simulink model "b_absorption_chiller_Yazaki_WFC_SC5_R2012a"  (Simulink 7.6)
settings: Solver=ode45  StartTime=0.0  StopTime=5000  FixedStep=1  RelTol=1e-3
PreLoadFcn:
  | load Yazaki_KF.mat;
values from neighbouring files (symbols this model uses):
  WFC_q_cold = [7.01442779481 14.9293699635 19.0103 4.77399164271 12.8469320096 16.2646 2.68674680792 10.4033145599 13.7100752403 6.86044435277 15.261380912 20.4077 ... (27 elements, 3x3x3)]    [Yazaki_KF.mat]
  WFC_q_hot = [11.58810793 12.70101443 13.76292339 14.78464775 15.7778999 16.75684251 17.73693962 18.73523022 19.7725001 20.87266321 21.46134147 22.12214918 ... (171 elements, 19x3x3)]    [Yazaki_KF.mat]
  WFC_q_recooling = [17.7490465324 34.7262277405 45.9087 12.9282238624 30.2579685905 40.8416 8.70035517453 25.0503537415 35.7528254726 17.2271014606 35.4257858178 48.632 ... (27 elements, 3x3x3)]    [Yazaki_KF.mat]
undefined symbols (not defined in the file or in its folder): A, B, C, Dd
settings Model: Creator=Simulation  LastModifiedBy=fabian.ille
settings DebuggingCC: FcnCallInpInsideContextMsg=Enable All
settings GRTTargetCC: CombineOutputUpdateFcns=on

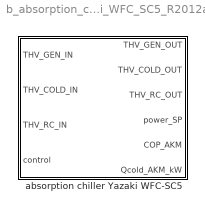
== system b_absorption_chiller_Yazaki_WFC_SC5_R2012a ==
  absorption chiller Yazaki WFC-SC5 : Subsystem
      mask Type: absorption chiller Yazaki WFC-SC5
      mask Description:
      | This block calculates the capacities and cop of the absorption chiller Yazaki WFC-SC5 (nominal cooling capacity: 17.6 kW, nominal COP: 0.7) based on measured curves.
      | Measurement range:
      | T_HT_IN 70 .. 88 °C, T_MT_IN 29 .. 33 °C, T_NT_IN 11 .. 14 °C
      | Outside of this range the lookup-tables extrapolate.
      | 
      | It is only valid for the following volumeflows:
      | HT: 4320 l/h, MT: 9180 l/h, NT: 2770 l/h
      | 
      | It includes a dynamic start-up behaviour with a dead time of the cooling capacity and capacities in all cycles.
      | Additionally the power of the solution pump is given out.
      mask Help: eval('helpcarnot')

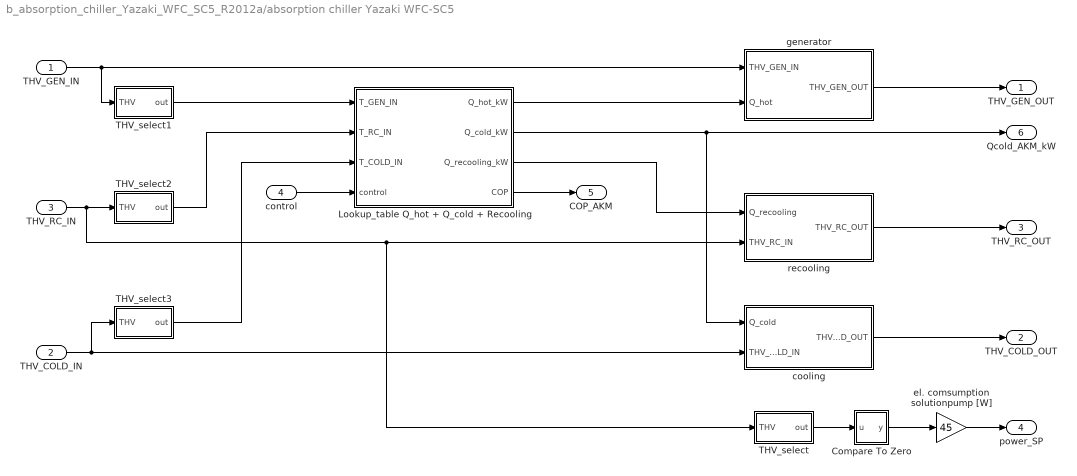
== system b_absorption_chiller_Yazaki_WFC_SC5_R2012a/absorption chiller Yazaki WFC-SC5 ==
  THV_GEN_IN : Inport
  THV_COLD_IN : Inport  Port=2
  THV_RC_IN : Inport  Port=3
  control : Inport  Port=4
  Compare To Zero : Subsystem  mask(Compare To Zero){relop=>, LogicOutDataTypeMode=uint8, ZeroCross=on}
      mask prompts: relop "Operator:"; LogicOutDataTypeMode "Output data type mode:"; ZeroCross "Enable zero-crossing detection"
      mask help: Determine how a signal compares to zero.
      mask init:
      | blkName = gcb;
      | 
      | if strcmp(get_param(gcbh,'LogicOutDataTypeMode'),'boolean')
      | 	setValue = 'Boolean';
      | else
      |     setValue = 'Specify via dialog';
      | end
      | 
      | set_param([blkName,'/Compare'],'relop',relop, ...
      | 	'LogicOutDataTypeMode', setValue, 'ZeroCross', ZeroCross);
      mask StyleString: popup(==|~=|<|<=|>=|>),popup(uint8|boolean),checkbox
      mask CallbackString: ||sl('zeroCrossEnable', gcbh);
      mask Display: disp([relop,' 0'])
  Lookup_table Q_hot + Q_cold + Recooling : Subsystem  TreatAsAtomicUnit=on
  THV_select : Subsystem  mask(select from THV){f=off, t=off, m=on, p=off, id=off, mix=off, d=off, dpcon=off, dplin=off, dpqua=off}
      mask prompts: f "flow identifier"; t "temperature [degree centigrade]"; m "massflow [kg/s]"; p "pressure [Pa]"; id "fluid ID (1 = water, 2 = air, 3 = cotton oil, 4 = water-glycol)"; mix "fluid mix"; d "diameter [m]"; dpcon "constant press. drop"; dplin "linear pressure drop"; dpqua "quadratic pressure drop"
      mask help: Selects the ticked values from the thermo hydraulic vector.
      mask init:
      | v=[];
      | if (f)
      |     v  = [1];
      | end
      | if (t)
      |     v  = [v 2];
      | end
      | if (m)
      |     v= [v 3];
      | end
      | if (p)
      |     v = [v 4];
      | end
      | if (id)
      |     v = [v 5];
      | end
      | if (mix)
      |     v = [v 6];
      | end
      | if (d)
      |     v = [v 7];
      | end
      | if (dpcon)
      |     v = [v 8];
      | end
      | if (dplin)
      |     v = [v 9];
      | end
      | if (dpqua)
      |     v = [v 10];
      | end
      mask Help: eval('man(''THV_select'')')
  THV_select1 : Subsystem  mask(select from THV){f=off, t=on, m=off, p=off, id=off, mix=off, d=off, dpcon=off, dplin=off, dpqua=off}
      mask prompts: f "flow identifier"; t "temperature [degree centigrade]"; m "massflow [kg/s]"; p "pressure [Pa]"; id "fluid ID (1 = water, 2 = air, 3 = cotton oil, 4 = water-glycol)"; mix "fluid mix"; d "diameter [m]"; dpcon "constant press. drop"; dplin "linear pressure drop"; dpqua "quadratic pressure drop"
      mask help: Selects the ticked values from the thermo hydraulic vector.
      mask init: same as b_absorption_chiller_Yazaki_WFC_SC5_R2012a/absorption chiller Yazaki WFC-SC5/THV_select
      mask Help: eval('man(''THV_select'')')
  THV_select2 : Subsystem  mask(select from THV){f=off, t=on, m=off, p=off, id=off, mix=off, d=off, dpcon=off, dplin=off, dpqua=off}
      mask prompts: f "flow identifier"; t "temperature [degree centigrade]"; m "massflow [kg/s]"; p "pressure [Pa]"; id "fluid ID (1 = water, 2 = air, 3 = cotton oil, 4 = water-glycol)"; mix "fluid mix"; d "diameter [m]"; dpcon "constant press. drop"; dplin "linear pressure drop"; dpqua "quadratic pressure drop"
      mask help: Selects the ticked values from the thermo hydraulic vector.
      mask init: same as b_absorption_chiller_Yazaki_WFC_SC5_R2012a/absorption chiller Yazaki WFC-SC5/THV_select
      mask Help: eval('man(''THV_select'')')
  THV_select3 : Subsystem  mask(select from THV){f=off, t=on, m=off, p=off, id=off, mix=off, d=off, dpcon=off, dplin=off, dpqua=off}
      mask prompts: f "flow identifier"; t "temperature [degree centigrade]"; m "massflow [kg/s]"; p "pressure [Pa]"; id "fluid ID (1 = water, 2 = air, 3 = cotton oil, 4 = water-glycol)"; mix "fluid mix"; d "diameter [m]"; dpcon "constant press. drop"; dplin "linear pressure drop"; dpqua "quadratic pressure drop"
      mask help: Selects the ticked values from the thermo hydraulic vector.
      mask init: same as b_absorption_chiller_Yazaki_WFC_SC5_R2012a/absorption chiller Yazaki WFC-SC5/THV_select
      mask Help: eval('man(''THV_select'')')
  cooling : Subsystem
  el. comsumption solutionpump [W] : Gain  Gain=45
  generator : Subsystem
  recooling : Subsystem
  THV_GEN_OUT : Outport
  THV_COLD_OUT : Outport  Port=2
  THV_RC_OUT : Outport  Port=3
  power_SP : Outport  Port=4
  COP_AKM : Outport  Port=5
  Qcold_AKM_kW : Outport  Port=6
  wires:
  THV_COLD_IN/1 -> THV_select3/1(THV), cooling/2(THV_COLD_IN)
  THV_GEN_IN/1 -> THV_select1/1(THV), generator/1(THV_GEN_IN)
  generator/1(THV_GEN_OUT) -> THV_GEN_OUT/1
  THV_RC_IN/1 -> THV_select2/1(THV), THV_select/1(THV), recooling/2(THV_RC_IN)
  THV_select2/1(out) -> Lookup_table Q_hot + Q_cold + Recooling/2(T_RC_IN)
  recooling/1(THV_RC_OUT) -> THV_RC_OUT/1
  cooling/1(THV_COLD_OUT) -> THV_COLD_OUT/1
  control/1 -> Lookup_table Q_hot + Q_cold + Recooling/4(control)
  THV_select3/1(out) -> Lookup_table Q_hot + Q_cold + Recooling/3(T_COLD_IN)
  Lookup_table Q_hot + Q_cold + Recooling/2(Q_cold_kW) -> cooling/1(Q_cold), Qcold_AKM_kW/1
  Lookup_table Q_hot + Q_cold + Recooling/1(Q_hot_kW) -> generator/2(Q_hot)
  Lookup_table Q_hot + Q_cold + Recooling/3(Q_recooling_kW) -> recooling/1(Q_recooling)
  el. comsumption solutionpump [W]/1 -> power_SP/1
  THV_select/1(out) -> Compare To Zero/1(u)
  Compare To Zero/1(y) -> el. comsumption solutionpump [W]/1
  THV_select1/1(out) -> Lookup_table Q_hot + Q_cold + Recooling/1(T_GEN_IN)
  Lookup_table Q_hot + Q_cold + Recooling/4(COP) -> COP_AKM/1

== system b_absorption_chiller_Yazaki_WFC_SC5_R2012a/absorption chiller Yazaki WFC-SC5/Compare To Zero ==
  u : Inport
  Compare : RelationalOperator  Operator=>  OutDataTypeStr=fixdt(0, 8)
  Constant : Constant  DisableCoverage=on  Value=0  OutDataTypeStr=Inherit: Inherit via back propagation  PreserveConstantTs=on
  y : Outport
  wires:
  Constant/1 -> Compare/2
  u/1 -> Compare/1
  Compare/1 -> y/1

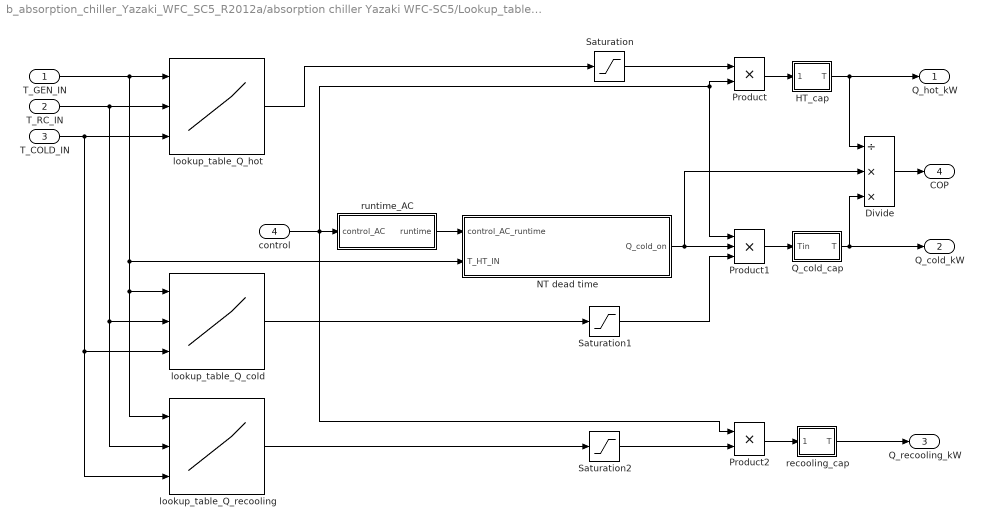
== system b_absorption_chiller_Yazaki_WFC_SC5_R2012a/absorption chiller Yazaki WFC-SC5/Lookup_table Q_hot + Q_cold + Recooling ==
  T_GEN_IN : Inport
  T_RC_IN : Inport  Port=2
  T_COLD_IN : Inport  Port=3
  control : Inport  Port=4
  Divide : Product  Inputs=/**
  HT_cap : Subsystem  mask(capacity){NTU=0.0464, Tini=0}
      mask prompts: NTU "heat transfer / heat capacity NTU (k*A/(m*cp))"; Tini "initial temperature [degree centigrade]"
      mask help: The block introduces a capacity of the component. It can be used to break an algebraic loop.
      mask Help: eval('man(''capacity'')')
  NT dead time : Stateflow chart  TreatAsAtomicUnit=on
  Product : Product  RndMeth=Zero
  Product1 : Product  Inputs=3  RndMeth=Zero
  Product2 : Product  RndMeth=Zero
  Q_cold_cap : Subsystem  mask(capacity){NTU=0.0191, Tini=0}
      mask prompts: NTU "heat transfer / heat capacity NTU (k*A/(m*cp))"; Tini "initial temperature [degree centigrade]"
      mask help: The block introduces a capacity of the component. It can be used to break an algebraic loop.
      mask Help: eval('man(''capacity'')')
  Saturation : Saturate  UpperLimit=inf  LowerLimit=0
  Saturation1 : Saturate  UpperLimit=inf  LowerLimit=0
  Saturation2 : Saturate  UpperLimit=inf  LowerLimit=0
  lookup_table_Q_cold : Lookup_n-D  NumberOfTableDimensions=3  BreakpointsForDimension1=[70,79,88]  BreakpointsForDimension2=[29,31,33]  BreakpointsForDimension3=[11,12.5,14]  BreakpointsForDimension4=[1:2]  Table=WFC_q_cold  InputSameDT=on
  lookup_table_Q_hot : Lookup_n-D  NumberOfTableDimensions=3  BreakpointsForDimension1=[70:1:88]  BreakpointsForDimension2=[29,31,33]  BreakpointsForDimension3=[11,12.5,14]  BreakpointsForDimension4=[1:2]  Table=WFC_q_hot  InputSameDT=on
  lookup_table_Q_recooling : Lookup_n-D  NumberOfTableDimensions=3  BreakpointsForDimension1=[70,79,88]  BreakpointsForDimension2=[29,31,33]  BreakpointsForDimension3=[11,12.5,14]  BreakpointsForDimension4=[1:2]  Table=WFC_q_recooling  InputSameDT=on
  recooling_cap : Subsystem  mask(capacity){NTU=0.0096, Tini=0}
      mask prompts: NTU "heat transfer / heat capacity NTU (k*A/(m*cp))"; Tini "initial temperature [degree centigrade]"
      mask help: The block introduces a capacity of the component. It can be used to break an algebraic loop.
      mask Help: eval('man(''capacity'')')
  runtime_AC : Subsystem  TreatAsAtomicUnit=on
      mask Description: This block counts the time if input is set to one, it stops counting if input is zero and continues when input rises to one again.
      mask Help: eval('filetest (''manual.htm#count_working_time'')')
  Q_hot_kW : Outport
  Q_cold_kW : Outport  Port=2
  Q_recooling_kW : Outport  Port=3
  COP : Outport  Port=4
  wires:
  T_COLD_IN/1 -> lookup_table_Q_cold/3, lookup_table_Q_recooling/3, lookup_table_Q_hot/3
  T_RC_IN/1 -> lookup_table_Q_cold/2, lookup_table_Q_recooling/2, lookup_table_Q_hot/2
  T_GEN_IN/1 -> NT dead time/2(T_HT_IN), lookup_table_Q_cold/1, lookup_table_Q_recooling/1, lookup_table_Q_hot/1
  lookup_table_Q_hot/1 -> Saturation/1
  control/1 -> runtime_AC/1(control_AC), Product/2, Product1/1, Product2/1
  runtime_AC/1(runtime) -> NT dead time/1(control_AC_runtime)
  Product/1 -> HT_cap/1(Tin)
  Product1/1 -> Q_cold_cap/1(Tin)
  HT_cap/1(T) -> Q_hot_kW/1, Divide/1
  Q_cold_cap/1(T) -> Q_cold_kW/1, Divide/3
  lookup_table_Q_cold/1 -> Saturation1/1
  recooling_cap/1(T) -> Q_recooling_kW/1
  Product2/1 -> recooling_cap/1(Tin)
  lookup_table_Q_recooling/1 -> Saturation2/1
  Saturation/1 -> Product/1
  Saturation1/1 -> Product1/3
  Saturation2/1 -> Product2/2
  Divide/1 -> COP/1
  NT dead time/1(Q_cold_on) -> Product1/2, Divide/2

== system b_absorption_chiller_Yazaki_WFC_SC5_R2012a/absorption chiller Yazaki WFC-SC5/THV_select ==
  THV : Inport
  Selector : Selector  InputPortWidth=20  IndexOptions=Index vector (dialog)  Indices=[v]  OutputSizes=1
  out : Outport  InitialOutput=0
  wires:
  THV/1 -> Selector/1
  Selector/1 -> out/1

== system b_absorption_chiller_Yazaki_WFC_SC5_R2012a/absorption chiller Yazaki WFC-SC5/THV_select1 ==
  THV : Inport
  Selector : Selector  InputPortWidth=20  IndexOptions=Index vector (dialog)  Indices=[v]  OutputSizes=1
  out : Outport  InitialOutput=0
  wires:
  THV/1 -> Selector/1
  Selector/1 -> out/1

== system b_absorption_chiller_Yazaki_WFC_SC5_R2012a/absorption chiller Yazaki WFC-SC5/THV_select2 ==
  THV : Inport
  Selector : Selector  InputPortWidth=20  IndexOptions=Index vector (dialog)  Indices=[v]  OutputSizes=1
  out : Outport  InitialOutput=0
  wires:
  THV/1 -> Selector/1
  Selector/1 -> out/1

== system b_absorption_chiller_Yazaki_WFC_SC5_R2012a/absorption chiller Yazaki WFC-SC5/THV_select3 ==
  THV : Inport
  Selector : Selector  InputPortWidth=20  IndexOptions=Index vector (dialog)  Indices=[v]  OutputSizes=1
  out : Outport  InitialOutput=0
  wires:
  THV/1 -> Selector/1
  Selector/1 -> out/1

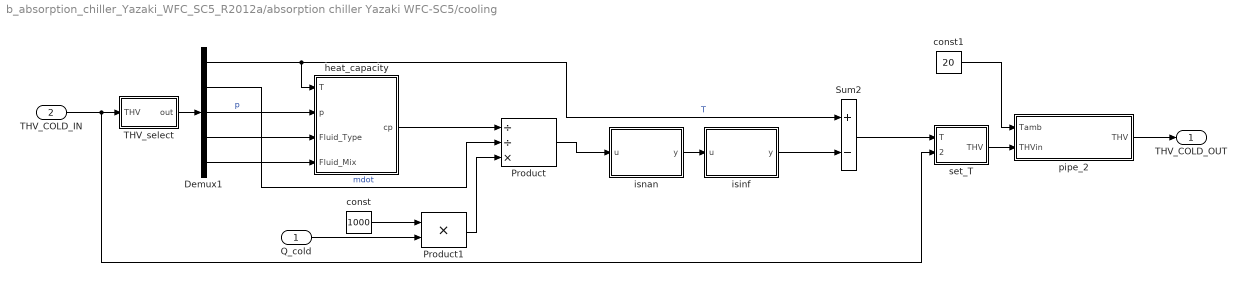
== system b_absorption_chiller_Yazaki_WFC_SC5_R2012a/absorption chiller Yazaki WFC-SC5/cooling ==
  Q_cold : Inport
  THV_COLD_IN : Inport  Port=2
  Demux1 : Demux  Outputs=5
  Product : Product  Inputs=//*  SaturateOnIntegerOverflow=on  RndMeth=Zero  InputSameDT=on  OutDataTypeStr=Inherit: Same as first input
  Product1 : Product  Inputs=**  SaturateOnIntegerOverflow=on  RndMeth=Zero  InputSameDT=on  OutDataTypeStr=Inherit: Same as first input
  Sum2 : Sum  Inputs=+-  InputSameDT=on  OutDataTypeStr=Inherit: Same as first input
  THV_select : Subsystem  mask(select from THV){f=off, t=on, m=on, p=on, id=on, mix=on, d=off, dpcon=off, dplin=off, dpqua=off}
      mask prompts: f "flow identifier"; t "temperature [degree centigrade]"; m "massflow [kg/s]"; p "pressure [Pa]"; id "fluid ID (1 = water, 2 = air, 3 = cotton oil, 4 = water-glycol)"; mix "fluid mix"; d "diameter [m]"; dpcon "constant press. drop"; dplin "linear pressure drop"; dpqua "quadratic pressure drop"
      mask help: Selects the ticked values from the thermo hydraulic vector.
      mask init: same as b_absorption_chiller_Yazaki_WFC_SC5_R2012a/absorption chiller Yazaki WFC-SC5/THV_select
      mask Help: eval('man(''THV_select'')')
  const : Constant  Value=1000
  const1 : Constant  Value=20
  heat_capacity : Subsystem
      mask Type: heat capacity
      mask Description:
      | Calculates the  heat_capacity of fluids [J/(kg*K)].
      | Calls calls the function "hcap" in the CARNOT library "carlib".
      | Definition of the fluid types
      | fluid-ID  material           remarks on fluid mix
      | 1           water              vapourcontent in the 2-phase region
      | 2           air                   is (kg water) / (kg air)
      | 3           cotton oil
      | 4           silicone oil
      | 5           water-glycol    gives the volume partition [0..1] of glycol
      | 6           tyfocor LS      only available in liquid phase
      mask Help: eval('man(''heat_capacity'')')
  isinf : Stateflow chart  TreatAsAtomicUnit=on
  isnan : Stateflow chart  TreatAsAtomicUnit=on
  pipe_2 : Subsystem  mask(pipe 2){d=0.029, l=12.2, uloss=0, cond=0, cwall=0, t0=20, nodes=5, dplin=0, dpqua=0, h=0}
      mask prompts: d "diameter [m]"; l "length of pipe [m]"; uloss "heat loss coefficient [W/(m²*K)]"; cond "effective conductivity in the pipe [W/(m*K)]"; cwall "capacity of pipewall per length in [J/(m*K)]"; t0 "initial temperature [degree centigrade]"; nodes "number of nodes"; dplin "pressure drop linear in massflow [Pa*s/kg]"; dpqua "pressure drop quadratic in massflow [Pa*s²/kg²]"; h "height [m], + for outlet above (0 for pump systems)"
      mask help:
      | Multinode pipe with capacity and easy pressure drop calculation. The pressure drop is a quadratic function of the massflow. The dependance of the quadratic term on the Reynolds number is neglected. The flow is calculated by the upwind scheme heat conduction between nodes by central differences (Patankar 1980).
      | heat loss: u = conductivity / ( d_in * ln (d_out / d_in) )
      mask init:
      | d = max(d, 0.0001);
      | l = max(l, 0.001);
      | cwall = max(0.001, cwall);
      | nodes = max(nodes, 1);
      mask Help: eval('man(''pipe_2'')')
      mask Display: plot(0,0,100,100,[24,27,27,24,75,80,80,75,24,20,20,24],[60,53,46,40,40,46,55,60,60,53,46,40])
  set_T : Subsystem
      mask Type: set temperature in THV
      mask Description: Set the temperature in the thermo-hydraulic vector.
      mask Help: eval('man(''set_T'')')
  THV_COLD_OUT : Outport
  wires:
  heat_capacity/1(cp) -> Product/1
  THV_COLD_IN/1 -> THV_select/1(THV), set_T/2(THV_in)
  Demux1/1 -> heat_capacity/1(T), Sum2/1  "T"
  Demux1/3 -> heat_capacity/2(p)  "p"
  Demux1/4 -> heat_capacity/3(Fluid_Type)
  Demux1/5 -> heat_capacity/4(Fluid_Mix)
  Q_cold/1 -> Product1/2
  const/1 -> Product1/1
  Product1/1 -> Product/3
  isnan/1(y) -> isinf/1(u)
  Product/1 -> isnan/1(u)
  isinf/1(y) -> Sum2/2
  Demux1/2 -> Product/2  "mdot"
  Sum2/1 -> set_T/1(T)
  pipe_2/1(THV) -> THV_COLD_OUT/1
  set_T/1(THV) -> pipe_2/2(THVin)
  const1/1 -> pipe_2/1(Tamb)
  THV_select/1(out) -> Demux1/1

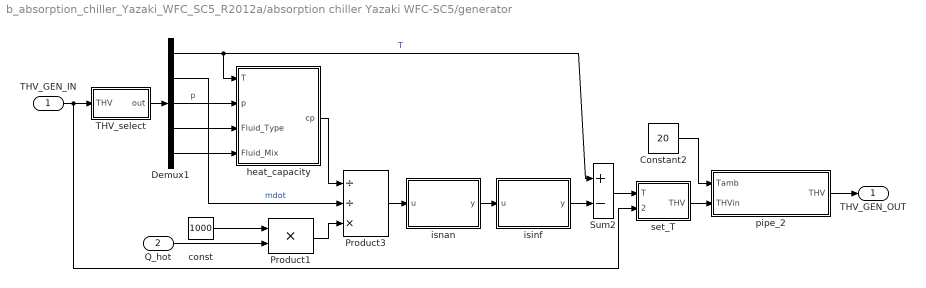
== system b_absorption_chiller_Yazaki_WFC_SC5_R2012a/absorption chiller Yazaki WFC-SC5/generator ==
  THV_GEN_IN : Inport
  Q_hot : Inport  Port=2
  Constant2 : Constant  Value=20
  Demux1 : Demux  Outputs=5
  Product1 : Product  Inputs=**  SaturateOnIntegerOverflow=on  RndMeth=Zero  InputSameDT=on  OutDataTypeStr=Inherit: Same as first input
  Product3 : Product  Inputs=//*  SaturateOnIntegerOverflow=on  RndMeth=Zero  InputSameDT=on  OutDataTypeStr=Inherit: Same as first input
  Sum2 : Sum  Inputs=+-  InputSameDT=on  OutDataTypeStr=Inherit: Same as first input
  THV_select : Subsystem  mask(select from THV){f=off, t=on, m=on, p=on, id=on, mix=on, d=off, dpcon=off, dplin=off, dpqua=off}
      mask prompts: f "flow identifier"; t "temperature [degree centigrade]"; m "massflow [kg/s]"; p "pressure [Pa]"; id "fluid ID (1 = water, 2 = air, 3 = cotton oil, 4 = water-glycol)"; mix "fluid mix"; d "diameter [m]"; dpcon "constant press. drop"; dplin "linear pressure drop"; dpqua "quadratic pressure drop"
      mask help: Selects the ticked values from the thermo hydraulic vector.
      mask init: same as b_absorption_chiller_Yazaki_WFC_SC5_R2012a/absorption chiller Yazaki WFC-SC5/THV_select
      mask Help: eval('man(''THV_select'')')
  const : Constant  Value=1000
  heat_capacity : Subsystem
      mask Type: heat capacity
      mask Description:
      | Calculates the  heat_capacity of fluids [J/(kg*K)].
      | Calls calls the function "hcap" in the CARNOT library "carlib".
      | Definition of the fluid types
      | fluid-ID  material           remarks on fluid mix
      | 1           water              vapourcontent in the 2-phase region
      | 2           air                   is (kg water) / (kg air)
      | 3           cotton oil
      | 4           silicone oil
      | 5           water-glycol    gives the volume partition [0..1] of glycol
      | 6           tyfocor LS      only available in liquid phase
      mask Help: eval('man(''heat_capacity'')')
  isinf : Stateflow chart  TreatAsAtomicUnit=on
  isnan : Stateflow chart  TreatAsAtomicUnit=on
  pipe_2 : Subsystem  mask(pipe 2){d=0.039, l=8.4, uloss=0, cond=0, cwall=0, t0=20, nodes=5, dplin=0, dpqua=0, h=0}
      mask prompts: d "diameter [m]"; l "length of pipe [m]"; uloss "heat loss coefficient [W/(m²*K)]"; cond "effective conductivity in the pipe [W/(m*K)]"; cwall "capacity of pipewall per length in [J/(m*K)]"; t0 "initial temperature [degree centigrade]"; nodes "number of nodes"; dplin "pressure drop linear in massflow [Pa*s/kg]"; dpqua "pressure drop quadratic in massflow [Pa*s²/kg²]"; h "height [m], + for outlet above (0 for pump systems)"
      mask help:
      | Multinode pipe with capacity and easy pressure drop calculation. The pressure drop is a quadratic function of the massflow. The dependance of the quadratic term on the Reynolds number is neglected. The flow is calculated by the upwind scheme heat conduction between nodes by central differences (Patankar 1980).
      | heat loss: u = conductivity / ( d_in * ln (d_out / d_in) )
      mask init:
      | d = max(d, 0.0001);
      | l = max(l, 0.001);
      | cwall = max(0.001, cwall);
      | nodes = max(nodes, 1);
      mask Help: eval('man(''pipe_2'')')
      mask Display: plot(0,0,100,100,[24,27,27,24,75,80,80,75,24,20,20,24],[60,53,46,40,40,46,55,60,60,53,46,40])
  set_T : Subsystem
      mask Type: set temperature in THV
      mask Description: Set the temperature in the thermo-hydraulic vector.
      mask Help: eval('man(''set_T'')')
  THV_GEN_OUT : Outport
  wires:
  Product3/1 -> isnan/1(u)
  Demux1/2 -> Product3/2  "mdot"
  heat_capacity/1(cp) -> Product3/1
  Demux1/3 -> heat_capacity/2(p)  "p"
  Demux1/5 -> heat_capacity/4(Fluid_Mix)
  Demux1/4 -> heat_capacity/3(Fluid_Type)
  Demux1/1 -> heat_capacity/1(T), Sum2/1  "T"
  Q_hot/1 -> Product1/2
  const/1 -> Product1/1
  Product1/1 -> Product3/3
  isnan/1(y) -> isinf/1(u)
  isinf/1(y) -> Sum2/2
  Sum2/1 -> set_T/1(T)
  set_T/1(THV) -> pipe_2/2(THVin)
  pipe_2/1(THV) -> THV_GEN_OUT/1
  Constant2/1 -> pipe_2/1(Tamb)
  THV_select/1(out) -> Demux1/1
  THV_GEN_IN/1 -> THV_select/1(THV), set_T/2(THV_in)

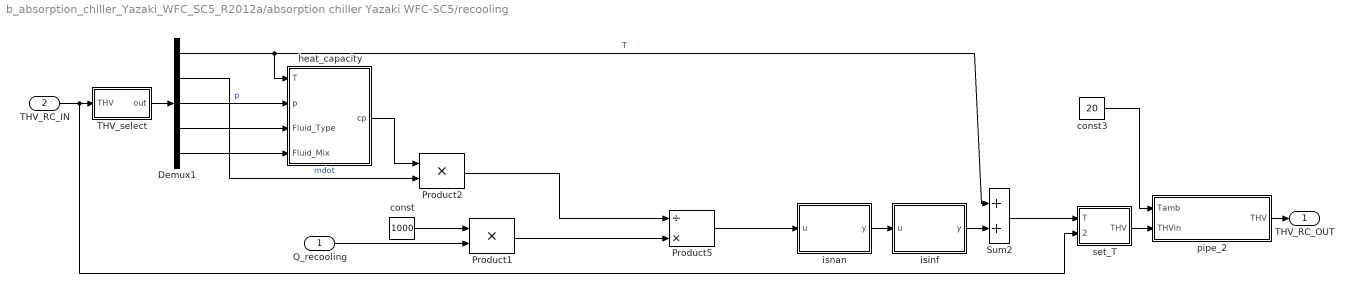
== system b_absorption_chiller_Yazaki_WFC_SC5_R2012a/absorption chiller Yazaki WFC-SC5/recooling ==
  Q_recooling : Inport
  THV_RC_IN : Inport  Port=2
  Demux1 : Demux  Outputs=5
  Product1 : Product  Inputs=**  SaturateOnIntegerOverflow=on  RndMeth=Zero  InputSameDT=on  OutDataTypeStr=Inherit: Same as first input
  Product2 : Product  Inputs=**  SaturateOnIntegerOverflow=on  RndMeth=Zero  InputSameDT=on  OutDataTypeStr=Inherit: Same as first input
  Product5 : Product  Inputs=/*  SaturateOnIntegerOverflow=on  RndMeth=Zero  InputSameDT=on  OutDataTypeStr=Inherit: Same as first input
  Sum2 : Sum  InputSameDT=on  OutDataTypeStr=Inherit: Same as first input
  THV_select : Subsystem  mask(select from THV){f=off, t=on, m=on, p=on, id=on, mix=on, d=off, dpcon=off, dplin=off, dpqua=off}
      mask prompts: f "flow identifier"; t "temperature [degree centigrade]"; m "massflow [kg/s]"; p "pressure [Pa]"; id "fluid ID (1 = water, 2 = air, 3 = cotton oil, 4 = water-glycol)"; mix "fluid mix"; d "diameter [m]"; dpcon "constant press. drop"; dplin "linear pressure drop"; dpqua "quadratic pressure drop"
      mask help: Selects the ticked values from the thermo hydraulic vector.
      mask init: same as b_absorption_chiller_Yazaki_WFC_SC5_R2012a/absorption chiller Yazaki WFC-SC5/THV_select
      mask Help: eval('man(''THV_select'')')
  const : Constant  Value=1000
  const3 : Constant  Value=20
  heat_capacity : Subsystem
      mask Type: heat capacity
      mask Description:
      | Calculates the  heat_capacity of fluids [J/(kg*K)].
      | Calls calls the function "hcap" in the CARNOT library "carlib".
      | Definition of the fluid types
      | fluid-ID  material           remarks on fluid mix
      | 1           water              vapourcontent in the 2-phase region
      | 2           air                   is (kg water) / (kg air)
      | 3           cotton oil
      | 4           silicone oil
      | 5           water-glycol    gives the volume partition [0..1] of glycol
      | 6           tyfocor LS      only available in liquid phase
      mask Help: eval('man(''heat_capacity'')')
  isinf : Stateflow chart  TreatAsAtomicUnit=on
  isnan : Stateflow chart  TreatAsAtomicUnit=on
  pipe_2 : Subsystem  mask(pipe 2){d=0.039, l=15.5, uloss=0, cond=0, cwall=0, t0=20, nodes=5, dplin=0, dpqua=0, h=0}
      mask prompts: d "diameter [m]"; l "length of pipe [m]"; uloss "heat loss coefficient [W/(m²*K)]"; cond "effective conductivity in the pipe [W/(m*K)]"; cwall "capacity of pipewall per length in [J/(m*K)]"; t0 "initial temperature [degree centigrade]"; nodes "number of nodes"; dplin "pressure drop linear in massflow [Pa*s/kg]"; dpqua "pressure drop quadratic in massflow [Pa*s²/kg²]"; h "height [m], + for outlet above (0 for pump systems)"
      mask help:
      | Multinode pipe with capacity and easy pressure drop calculation. The pressure drop is a quadratic function of the massflow. The dependance of the quadratic term on the Reynolds number is neglected. The flow is calculated by the upwind scheme heat conduction between nodes by central differences (Patankar 1980).
      | heat loss: u = conductivity / ( d_in * ln (d_out / d_in) )
      mask init:
      | d = max(d, 0.0001);
      | l = max(l, 0.001);
      | cwall = max(0.001, cwall);
      | nodes = max(nodes, 1);
      mask Help: eval('man(''pipe_2'')')
      mask Display: plot(0,0,100,100,[24,27,27,24,75,80,80,75,24,20,20,24],[60,53,46,40,40,46,55,60,60,53,46,40])
  set_T : Subsystem
      mask Type: set temperature in THV
      mask Description: Set the temperature in the thermo-hydraulic vector.
      mask Help: eval('man(''set_T'')')
  THV_RC_OUT : Outport
  wires:
  Product1/1 -> Product5/2
  Product2/1 -> Product5/1
  Demux1/2 -> Product2/2  "mdot"
  heat_capacity/1(cp) -> Product2/1
  Demux1/3 -> heat_capacity/2(p)  "p"
  Demux1/5 -> heat_capacity/4(Fluid_Mix)
  Demux1/4 -> heat_capacity/3(Fluid_Type)
  Demux1/1 -> heat_capacity/1(T), Sum2/1  "T"
  Q_recooling/1 -> Product1/2
  const/1 -> Product1/1
  isnan/1(y) -> isinf/1(u)
  isinf/1(y) -> Sum2/2
  Sum2/1 -> set_T/1(T)
  Product5/1 -> isnan/1(u)
  set_T/1(THV) -> pipe_2/2(THVin)
  pipe_2/1(THV) -> THV_RC_OUT/1
  const3/1 -> pipe_2/1(Tamb)
  THV_select/1(out) -> Demux1/1
  THV_RC_IN/1 -> THV_select/1(THV), set_T/2(THV_in)

== system b_absorption_chiller_Yazaki_WFC_SC5_R2012a/absorption chiller Yazaki WFC-SC5/Lookup_table Q_hot + Q_cold + Recooling/HT_cap ==
  Tin : Inport
  Transfer Fcn (with initial outputs) : Subsystem  mask(Transfer Function with Initial Outputs){N=[1], D=[1/NTU  1], Y0=Tini, U0=0}
      mask prompts: N "Numerator:"; D "Denominator:"; Y0 "Initial output:"; U0 "Initial input:"
      mask help: Vector expressions for numerator, and denominator. Coefficients are in descending powers of s.
      mask init:
      | [A,B,C,Dd]=tf2ss(N,D);
      | if (isempty(Y0));
      |     [m,n]=size(C);
      |     Y0=zeros(1,m); 
      | end; 
      | if (isempty(U0));
      |     [m,p]=size(B);
      |     U0=zeros(1,p);
      | end;
      | X0=getxo(A,B,C,Dd,U0,Y0,0);
      mask Help: Specify the initial output for the transfer function.  An optimization routine attempts to determine the appropriate initial states so that the specified initial output is achieved.  For more details, see the m-file getxo.m
      mask Display: dpoly(N,D,'s')
  T : Outport
  wires:
  Tin/1 -> Transfer Fcn (with initial outputs)/1(In1)
  Transfer Fcn (with initial outputs)/1(Out1) -> T/1

== system b_absorption_chiller_Yazaki_WFC_SC5_R2012a/absorption chiller Yazaki WFC-SC5/Lookup_table Q_hot + Q_cold + Recooling/Q_cold_cap ==
  Tin : Inport
  Transfer Fcn (with initial outputs) : Subsystem  mask(Transfer Function with Initial Outputs){N=[1], D=[1/NTU  1], Y0=Tini, U0=0}
      mask prompts: N "Numerator:"; D "Denominator:"; Y0 "Initial output:"; U0 "Initial input:"
      mask help: Vector expressions for numerator, and denominator. Coefficients are in descending powers of s.
      mask init:
      | [A,B,C,Dd]=tf2ss(N,D);
      | if (isempty(Y0));
      |     [m,n]=size(C);
      |     Y0=zeros(1,m); 
      | end; 
      | if (isempty(U0));
      |     [m,p]=size(B);
      |     U0=zeros(1,p);
      | end;
      | X0=getxo(A,B,C,Dd,U0,Y0,0);
      mask Help: Specify the initial output for the transfer function.  An optimization routine attempts to determine the appropriate initial states so that the specified initial output is achieved.  For more details, see the m-file getxo.m
      mask Display: dpoly(N,D,'s')
  T : Outport
  wires:
  Tin/1 -> Transfer Fcn (with initial outputs)/1(In1)
  Transfer Fcn (with initial outputs)/1(Out1) -> T/1

== system b_absorption_chiller_Yazaki_WFC_SC5_R2012a/absorption chiller Yazaki WFC-SC5/Lookup_table Q_hot + Q_cold + Recooling/recooling_cap ==
  Tin : Inport
  Transfer Fcn (with initial outputs) : Subsystem  mask(Transfer Function with Initial Outputs){N=[1], D=[1/NTU  1], Y0=Tini, U0=0}
      mask prompts: N "Numerator:"; D "Denominator:"; Y0 "Initial output:"; U0 "Initial input:"
      mask help: Vector expressions for numerator, and denominator. Coefficients are in descending powers of s.
      mask init:
      | [A,B,C,Dd]=tf2ss(N,D);
      | if (isempty(Y0));
      |     [m,n]=size(C);
      |     Y0=zeros(1,m); 
      | end; 
      | if (isempty(U0));
      |     [m,p]=size(B);
      |     U0=zeros(1,p);
      | end;
      | X0=getxo(A,B,C,Dd,U0,Y0,0);
      mask Help: Specify the initial output for the transfer function.  An optimization routine attempts to determine the appropriate initial states so that the specified initial output is achieved.  For more details, see the m-file getxo.m
      mask Display: dpoly(N,D,'s')
  T : Outport
  wires:
  Tin/1 -> Transfer Fcn (with initial outputs)/1(In1)
  Transfer Fcn (with initial outputs)/1(Out1) -> T/1

== system b_absorption_chiller_Yazaki_WFC_SC5_R2012a/absorption chiller Yazaki WFC-SC5/Lookup_table Q_hot + Q_cold + Recooling/runtime_AC ==
  control_AC : Inport
  Integrator : Integrator  ExternalReset=either
  runtime : Outport  InitialOutput=0
  wires:
  control_AC/1 -> Integrator/2, Integrator/1
  Integrator/1 -> runtime/1

== system b_absorption_chiller_Yazaki_WFC_SC5_R2012a/absorption chiller Yazaki WFC-SC5/cooling/THV_select ==
  THV : Inport
  Selector : Selector  InputPortWidth=20  IndexOptions=Index vector (dialog)  Indices=[v]  OutputSizes=1
  out : Outport  InitialOutput=0
  wires:
  THV/1 -> Selector/1
  Selector/1 -> out/1

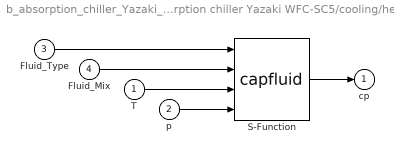
== system b_absorption_chiller_Yazaki_WFC_SC5_R2012a/absorption chiller Yazaki WFC-SC5/cooling/heat_capacity ==
  T : Inport
  p : Inport  Port=2
  Fluid_Type : Inport  Port=3
  Fluid_Mix : Inport  Port=4
  S-Function : S-Function  FunctionName=capfluid  EnableBusSupport=off
  cp : Outport  InitialOutput=0
  wires:
  S-Function/1 -> cp/1
  Fluid_Type/1 -> S-Function/1
  Fluid_Mix/1 -> S-Function/2
  T/1 -> S-Function/3
  p/1 -> S-Function/4

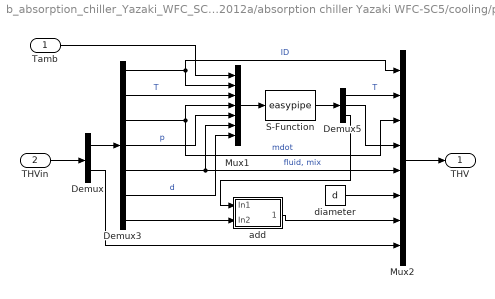
== system b_absorption_chiller_Yazaki_WFC_SC5_R2012a/absorption chiller Yazaki WFC-SC5/cooling/pipe_2 ==
  Tamb : Inport
  THVin : Inport  Port=2
  Demux : Demux  Outputs=[10 10]
  Demux3 : Demux  Outputs=[1 1 1 1 2 1 3]
  Demux5 : Demux  Outputs=3
  Mux1 : Mux  Inputs=7
  Mux2 : Mux  Inputs=8
  S-Function : S-Function  FunctionName=easypipe  Parameters="d, l,  uloss,  cond,  cwall,  t0, nodes, dplin, dpqua, h"  EnableBusSupport=off
  add : Subsystem
  diameter : Constant  Value=d
  THV : Outport  InitialOutput=0
  wires:
  Demux3/7 -> add/2(In2)
  add/1(Out1) -> Mux2/7
  Demux5/3 -> add/1(In1)
  Demux/2 -> Mux2/8
  THVin/1 -> Demux/1
  Demux/1 -> Demux3/1
  Demux3/1 -> Mux2/1, Mux1/2  "ID"
  Demux3/2 -> Mux1/3  "T"
  Demux3/6 -> Mux1/7  "d"
  Demux3/3 -> Mux1/4, Mux2/3  "mdot"
  Demux3/5 -> Mux1/6, Mux2/5  "fluid, mix"
  Demux3/4 -> Mux1/5  "p"
  Demux5/1 -> Mux2/2  "T"
  diameter/1 -> Mux2/6
  Mux2/1 -> THV/1
  Tamb/1 -> Mux1/1
  S-Function/1 -> Demux5/1
  Mux1/1 -> S-Function/1
  Demux5/2 -> Mux2/4

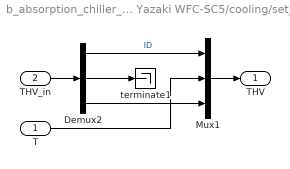
== system b_absorption_chiller_Yazaki_WFC_SC5_R2012a/absorption chiller Yazaki WFC-SC5/cooling/set_T ==
  T : Inport
  THV_in : Inport  Port=2
  Demux2 : Demux  Outputs=[1 1 18]
  Mux1 : Mux  Inputs=3
  terminate1 : Terminator
  THV : Outport  InitialOutput=0
  wires:
  Demux2/2 -> terminate1/1
  THV_in/1 -> Demux2/1
  Demux2/1 -> Mux1/1  "ID"
  Demux2/3 -> Mux1/3
  T/1 -> Mux1/2
  Mux1/1 -> THV/1

== system b_absorption_chiller_Yazaki_WFC_SC5_R2012a/absorption chiller Yazaki WFC-SC5/generator/THV_select ==
  THV : Inport
  Selector : Selector  InputPortWidth=20  IndexOptions=Index vector (dialog)  Indices=[v]  OutputSizes=1
  out : Outport  InitialOutput=0
  wires:
  THV/1 -> Selector/1
  Selector/1 -> out/1

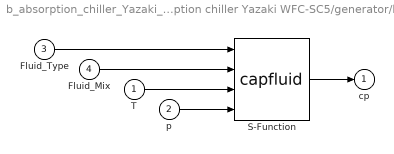
== system b_absorption_chiller_Yazaki_WFC_SC5_R2012a/absorption chiller Yazaki WFC-SC5/generator/heat_capacity ==
  T : Inport
  p : Inport  Port=2
  Fluid_Type : Inport  Port=3
  Fluid_Mix : Inport  Port=4
  S-Function : S-Function  FunctionName=capfluid  EnableBusSupport=off
  cp : Outport  InitialOutput=0
  wires:
  S-Function/1 -> cp/1
  Fluid_Type/1 -> S-Function/1
  Fluid_Mix/1 -> S-Function/2
  T/1 -> S-Function/3
  p/1 -> S-Function/4

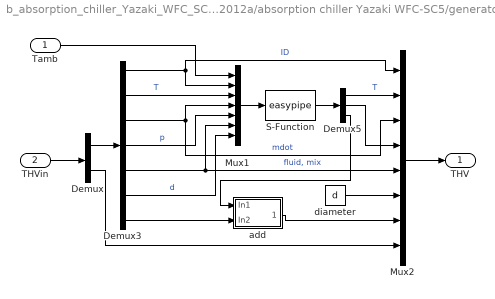
== system b_absorption_chiller_Yazaki_WFC_SC5_R2012a/absorption chiller Yazaki WFC-SC5/generator/pipe_2 ==
  Tamb : Inport
  THVin : Inport  Port=2
  Demux : Demux  Outputs=[10 10]
  Demux3 : Demux  Outputs=[1 1 1 1 2 1 3]
  Demux5 : Demux  Outputs=3
  Mux1 : Mux  Inputs=7
  Mux2 : Mux  Inputs=8
  S-Function : S-Function  FunctionName=easypipe  Parameters="d, l,  uloss,  cond,  cwall,  t0, nodes, dplin, dpqua, h"  EnableBusSupport=off
  add : Subsystem
  diameter : Constant  Value=d
  THV : Outport  InitialOutput=0
  wires:
  Demux3/7 -> add/2(In2)
  add/1(Out1) -> Mux2/7
  Demux5/3 -> add/1(In1)
  Demux/2 -> Mux2/8
  THVin/1 -> Demux/1
  Demux/1 -> Demux3/1
  Demux3/1 -> Mux2/1, Mux1/2  "ID"
  Demux3/2 -> Mux1/3  "T"
  Demux3/6 -> Mux1/7  "d"
  Demux3/3 -> Mux1/4, Mux2/3  "mdot"
  Demux3/5 -> Mux1/6, Mux2/5  "fluid, mix"
  Demux3/4 -> Mux1/5  "p"
  Demux5/1 -> Mux2/2  "T"
  diameter/1 -> Mux2/6
  Mux2/1 -> THV/1
  Tamb/1 -> Mux1/1
  S-Function/1 -> Demux5/1
  Mux1/1 -> S-Function/1
  Demux5/2 -> Mux2/4

== system b_absorption_chiller_Yazaki_WFC_SC5_R2012a/absorption chiller Yazaki WFC-SC5/generator/set_T ==
  T : Inport
  THV_in : Inport  Port=2
  Demux2 : Demux  Outputs=[1 1 18]
  Mux1 : Mux  Inputs=3
  terminate1 : Terminator
  THV : Outport  InitialOutput=0
  wires:
  Demux2/2 -> terminate1/1
  THV_in/1 -> Demux2/1
  Demux2/1 -> Mux1/1  "ID"
  Demux2/3 -> Mux1/3
  Mux1/1 -> THV/1
  T/1 -> Mux1/2

== system b_absorption_chiller_Yazaki_WFC_SC5_R2012a/absorption chiller Yazaki WFC-SC5/recooling/THV_select ==
  THV : Inport
  Selector : Selector  InputPortWidth=20  IndexOptions=Index vector (dialog)  Indices=[v]  OutputSizes=1
  out : Outport  InitialOutput=0
  wires:
  THV/1 -> Selector/1
  Selector/1 -> out/1

== system b_absorption_chiller_Yazaki_WFC_SC5_R2012a/absorption chiller Yazaki WFC-SC5/recooling/heat_capacity ==
  T : Inport
  p : Inport  Port=2
  Fluid_Type : Inport  Port=3
  Fluid_Mix : Inport  Port=4
  S-Function : S-Function  FunctionName=capfluid  EnableBusSupport=off
  cp : Outport  InitialOutput=0
  wires:
  S-Function/1 -> cp/1
  Fluid_Type/1 -> S-Function/1
  Fluid_Mix/1 -> S-Function/2
  T/1 -> S-Function/3
  p/1 -> S-Function/4

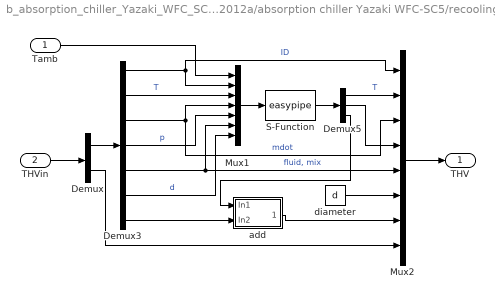
== system b_absorption_chiller_Yazaki_WFC_SC5_R2012a/absorption chiller Yazaki WFC-SC5/recooling/pipe_2 ==
  Tamb : Inport
  THVin : Inport  Port=2
  Demux : Demux  Outputs=[10 10]
  Demux3 : Demux  Outputs=[1 1 1 1 2 1 3]
  Demux5 : Demux  Outputs=3
  Mux1 : Mux  Inputs=7
  Mux2 : Mux  Inputs=8
  S-Function : S-Function  FunctionName=easypipe  Parameters="d, l,  uloss,  cond,  cwall,  t0, nodes, dplin, dpqua, h"  EnableBusSupport=off
  add : Subsystem
  diameter : Constant  Value=d
  THV : Outport  InitialOutput=0
  wires:
  Demux3/7 -> add/2(In2)
  add/1(Out1) -> Mux2/7
  Demux5/3 -> add/1(In1)
  Demux/2 -> Mux2/8
  THVin/1 -> Demux/1
  Demux/1 -> Demux3/1
  Demux3/1 -> Mux2/1, Mux1/2  "ID"
  Demux3/2 -> Mux1/3  "T"
  Demux3/6 -> Mux1/7  "d"
  Demux3/3 -> Mux1/4, Mux2/3  "mdot"
  Demux3/5 -> Mux1/6, Mux2/5  "fluid, mix"
  Demux3/4 -> Mux1/5  "p"
  Demux5/1 -> Mux2/2  "T"
  diameter/1 -> Mux2/6
  Mux2/1 -> THV/1
  Tamb/1 -> Mux1/1
  S-Function/1 -> Demux5/1
  Mux1/1 -> S-Function/1
  Demux5/2 -> Mux2/4

== system b_absorption_chiller_Yazaki_WFC_SC5_R2012a/absorption chiller Yazaki WFC-SC5/recooling/set_T ==
  T : Inport
  THV_in : Inport  Port=2
  Demux2 : Demux  Outputs=[1 1 18]
  Mux1 : Mux  Inputs=3
  terminate1 : Terminator
  THV : Outport  InitialOutput=0
  wires:
  Demux2/2 -> terminate1/1
  THV_in/1 -> Demux2/1
  Demux2/1 -> Mux1/1  "ID"
  Demux2/3 -> Mux1/3
  T/1 -> Mux1/2
  Mux1/1 -> THV/1

== system b_absorption_chiller_Yazaki_WFC_SC5_R2012a/absorption chiller Yazaki WFC-SC5/Lookup_table Q_hot + Q_cold + Recooling/HT_cap/Transfer Fcn (with initial outputs) ==
  In1 : Inport
  State Space : StateSpace  A=A  B=B  C=C  D=Dd  X0=X0
  Out1 : Outport  InitialOutput=0
  wires:
  State Space/1 -> Out1/1
  In1/1 -> State Space/1

== system b_absorption_chiller_Yazaki_WFC_SC5_R2012a/absorption chiller Yazaki WFC-SC5/Lookup_table Q_hot + Q_cold + Recooling/Q_cold_cap/Transfer Fcn (with initial outputs) ==
  In1 : Inport
  State Space : StateSpace  A=A  B=B  C=C  D=Dd  X0=X0
  Out1 : Outport  InitialOutput=0
  wires:
  State Space/1 -> Out1/1
  In1/1 -> State Space/1

== system b_absorption_chiller_Yazaki_WFC_SC5_R2012a/absorption chiller Yazaki WFC-SC5/Lookup_table Q_hot + Q_cold + Recooling/recooling_cap/Transfer Fcn (with initial outputs) ==
  In1 : Inport
  State Space : StateSpace  A=A  B=B  C=C  D=Dd  X0=X0
  Out1 : Outport  InitialOutput=0
  wires:
  State Space/1 -> Out1/1
  In1/1 -> State Space/1

== system b_absorption_chiller_Yazaki_WFC_SC5_R2012a/absorption chiller Yazaki WFC-SC5/cooling/pipe_2/add ==
  In1 : Inport
  In2 : Inport  Port=2
  Mux3 : Mux  Inputs=2
  Sum : Sum  SaturateOnIntegerOverflow=on  InputSameDT=on  OutDataTypeStr=Inherit: Same as first input
  const : Constant  Value=[dplin dpqua]
  Out1 : Outport  InitialOutput=0
  wires:
  In2/1 -> Sum/2
  Sum/1 -> Out1/1
  In1/1 -> Mux3/1
  Mux3/1 -> Sum/1
  const/1 -> Mux3/2

== system b_absorption_chiller_Yazaki_WFC_SC5_R2012a/absorption chiller Yazaki WFC-SC5/generator/pipe_2/add ==
  In1 : Inport
  In2 : Inport  Port=2
  Mux3 : Mux  Inputs=2
  Sum : Sum  SaturateOnIntegerOverflow=on  InputSameDT=on  OutDataTypeStr=Inherit: Same as first input
  const : Constant  Value=[dplin dpqua]
  Out1 : Outport  InitialOutput=0
  wires:
  In2/1 -> Sum/2
  Sum/1 -> Out1/1
  In1/1 -> Mux3/1
  Mux3/1 -> Sum/1
  const/1 -> Mux3/2

== system b_absorption_chiller_Yazaki_WFC_SC5_R2012a/absorption chiller Yazaki WFC-SC5/recooling/pipe_2/add ==
  In1 : Inport
  In2 : Inport  Port=2
  Mux3 : Mux  Inputs=2
  Sum : Sum  SaturateOnIntegerOverflow=on  InputSameDT=on  OutDataTypeStr=Inherit: Same as first input
  const : Constant  Value=[dplin dpqua]
  Out1 : Outport  InitialOutput=0
  wires:
  In2/1 -> Sum/2
  Sum/1 -> Out1/1
  In1/1 -> Mux3/1
  Mux3/1 -> Sum/1
  const/1 -> Mux3/2

== matlab function absorption chiller Yazaki WFC-SC5/cooling/isinf ==
  data: u input double; y output double

function y = fcn(u)

%Verhindert die Fehlerausgabe bei Teilen mit dem Wert 0 
%Dieser Zustand tritt ein wenn der Volumenstrom 0 l/s gesetzt wird.

v = isinf (u);

if v == 0
    
    y = u;

else 
    
    y = 0;
    
end

== matlab function absorption chiller Yazaki WFC-SC5/cooling/isnan ==
  data: u input double; y output double

function y = fcn(u)

%Verhindert die Fehlerausgabe bei Teilen durch den Wert 0 
%Dieser Zustand tritt ein wenn der Volumenstrom 0 l/s gesetzt wird.

v = isnan (u);

if v == 0
    
    y = u;

else 
    
    y = 0;
    
end

== stateflow chart absorption chiller Yazaki WFC-SC5/Lookup_table Q_hot + Q_cold + Recooling/NT dead time ==
  state request
    en:NT_dead_time=0;
    en:Q_cold_on=0;
  state calculation
    en:NT_dead_time=11768*T_HT_IN^(-1.205);
  state comparison
    en:Q_cold_on=1;
  (default) -> request
  request -> calculation : [(control_AC_runtime>=1)]
  calculation -> request [order 1] : [(control_AC_runtime==0)]
  calculation -> comparison [order 2] : [(control_AC_runtime>=NT_dead_time)]
  comparison -> request : [(control_AC_runtime==0)]
  data: control_AC_runtime input double; T_HT_IN input double; NT_dead_time local double; Q_cold_on output double

== matlab function absorption chiller Yazaki WFC-SC5/generator/isinf ==
  data: u input double; y output double

function y = fcn(u)

%Verhindert die Fehlerausgabe bei Teilen mit dem Wert 0 
%Dieser Zustand tritt ein wenn der Volumenstrom 0 l/s gesetzt wird.

v = isinf (u);

if v == 0
    
    y = u;

else 
    
    y = 0;
    
end

== matlab function absorption chiller Yazaki WFC-SC5/generator/isnan ==
  data: u input double; y output double

function y = fcn(u)

%Verhindert die Fehlerausgabe bei Teilen durch den Wert 0 
%Dieser Zustand tritt ein wenn der Volumenstrom 0 l/s gesetzt wird.

v = isnan (u);

if v == 0
    
    y = u;

else 
    
    y = 0;
    
end

== matlab function absorption chiller Yazaki WFC-SC5/recooling/isinf ==
  data: u input double; y output double

function y = fcn(u)

%Verhindert die Fehlerausgabe bei Teilen mit dem Wert 0 
%Dieser Zustand tritt ein wenn der Volumenstrom 0 l/s gesetzt wird.

v = isinf (u);

if v == 0
    
    y = u;

else 
    
    y = 0;
    
end

== matlab function absorption chiller Yazaki WFC-SC5/recooling/isnan ==
  data: u input double; y output double

function y = fcn(u)

%Verhindert die Fehlerausgabe bei Teilen durch den Wert 0 
%Dieser Zustand tritt ein wenn der Volumenstrom 0 l/s gesetzt wird.

v = isnan (u);

if v == 0
    
    y = u;

else 
    
    y = 0;
    
end
